simulink model "identifica_ip02"  (Simulink 7.2)
settings: Solver=ode4  StartTime=0.0  StopTime=10  FixedStep=0.001  RelTol=1e-3  AbsTol=1e-6
values from neighbouring files (symbols this model uses):
  Beq = 5.4    [matlab.mat]    (also in matlab2.mat)
  Eff_g = 1    [matlab.mat]    (also in matlab2.mat)
  Eff_m = 1    [matlab.mat]    (also in matlab2.mat)
  IMAX_AMP = 4    [matlab.mat]    (also in matlab2.mat)
  Jm = 3.90009575504e-07    [matlab.mat]    (also in matlab2.mat)
  K = yfinal*wn^2/amp_step    [estima_sys_2ordem.m]    (also in matlab.mat = 1; matlab2.mat = 1)
  K_AMP = 1    [matlab.mat]    (also in matlab2.mat)
  K_EC = 2.27485440932e-05    [matlab.mat]    (also in matlab2.mat)
  K_EP = 0.00153398078789    [matlab.mat]    (also in matlab2.mat)
  Kg = 3.71    [matlab.mat]    (also in matlab2.mat)
  Km = 0.00767763445475    [matlab.mat]    (also in matlab2.mat)
  Kt = 0.00768296972928    [matlab.mat]    (also in matlab2.mat)
  M = 0.94    [matlab.mat]    (also in matlab2.mat)
  qsi = -log(SP/100)/sqrt(pi^2+log(SP/100)^2)    [estima_sys_2ordem.m]    (also in matlab.mat = 1; matlab2.mat = 1)
  r_mp = 0.00635    [matlab.mat]    (also in matlab2.mat)
  R_SLEW_RATE = 500    [matlab.mat]    (also in matlab2.mat)
  Rm = 2.6    [matlab.mat]    (also in matlab2.mat)
  VMAX_AMP = 24    [matlab.mat]    (also in matlab2.mat)
  VMAX_DAC = 10    [matlab.mat]    (also in matlab2.mat)
  wn = pi/(Tp*sqrt(1-qsi^2))    [estima_sys_2ordem.m]    (also in identificacao.m = pi/(tp*sqrt(1-ksi^2)); matlab.mat = 1; matlab2.mat = 1)
  X_LIM_ENABLE = 1    [matlab.mat]    (also in matlab2.mat)
  X_MAX = 0.3    [matlab.mat]    (also in matlab2.mat)
  X_MIN = -0.3    [matlab.mat]    (also in matlab2.mat)
undefined symbols (not defined in the file or in its folder): HIL, qc_get_step_size
libraries: quarc_library x5, simulink x2, simulink_extras x1
CloseFcn:
  | rtwprivate ssgencode ModelCloseRequest q_position_pv_ip02
settings Model: Creator=Mfotoohi  LastModifiedBy=aluno  SimulationMode=external  ExtModeTrigDuration=50000  BufferReuse=off
settings SolverCC: PositivePriorityOrder=on
settings DataIOCC: LimitDataPoints=off
settings OptimizationCC: BooleanDataType=off  InlineInvariantSignals=on  OptimizeBlockIOStorage=off  BufferReuse=off  EnforceIntegerDowncast=off  ExpressionFolding=off  FoldNonRolledExpr=off  LocalBlockOutputs=off  InitFltsAndDblsToZero=on
settings DebuggingCC: SaveWithParameterizedLinksMsg=none  SignalResolutionControl=TryResolveAllWithWarning  SolverPrmCheckMsg=none  MultiTaskDSMMsg=warning  MultiTaskCondExecSysMsg=none  StrictBusMsg=None
settings HardwareCC: TargetHWDeviceType=32-bit Generic
settings RTWCC: SystemTargetFile=quarc_windows.tlc  TemplateMakefile=quarc_default_tmf  Description=Quarc Win32 Target  ProcessScript=quarc_windows_make_rtw_hook  IncludeERTFirstTime=on
settings STFCustomTargetCC: TargetFcnLib=ansi_tfl_tmw.mat  TargetPreCompLibLocation=C:\DOCUME~1\ALLUSE~1\DADOSD~1\QUARC\lib\2008b\windows\release  SystemTargetFile=quarc_windows.tlc
settings GRTTargetCC: TargetFcnLib=ansi_tfl_tmw.mat  TargetPreCompLibLocation=C:\DOCUME~1\ALLUSE~1\DADOSD~1\QUARC\lib\2008b\windows\release  CompOptLevelCompliant=off  MatFileLogging=off  ExtMode=on  ExtModeMexFile=quarc_comm

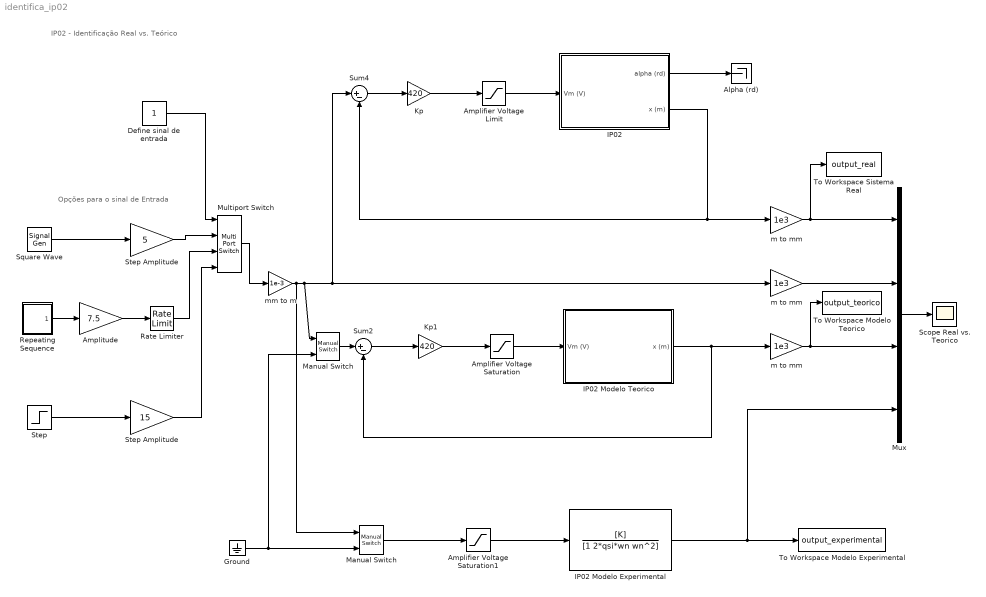
== system identifica_ip02 ==
  note: IP02 - Identificação
      | Real vs. Teórico
  note: Opções para o sinal de Entrada
  Alpha (rd) : Terminator
  Amplifier Voltage Limit : Saturate  UpperLimit=VMAX_AMP  LowerLimit=- VMAX_AMP
  Amplifier Voltage Saturation : Saturate  UpperLimit=VMAX_AMP  LowerLimit=- VMAX_AMP
  Amplifier Voltage Saturation1 : Saturate  UpperLimit=VMAX_AMP  LowerLimit=- VMAX_AMP
  Amplitude : Gain  Gain=7.5  ParameterDataType=sfix(16)  ParameterScaling=2^0  OutDataType=sfix(16)  OutScaling=2^0  SaturateOnIntegerOverflow=on  OutDataTypeStr=Inherit: Same as input  ParamDataTypeStr=Inherit: Same as input
  Define sinal de entrada : Constant  OutDataType=fixdt(1, 16)  OutScaling=2^0
  Ground : Ground
  IP02 : Subsystem
  IP02 Modelo Experimental : TransferFcn  Numerator=[K]  Denominator=[1 2*qsi*wn wn^2]
  IP02 Modelo Teorico : Subsystem
  Kp : Gain  Gain=420  ParameterDataType=sfix(16)  ParameterScaling=2^0  OutDataType=sfix(16)  OutScaling=2^0  SaturateOnIntegerOverflow=on  OutDataTypeStr=Inherit: Same as input  ParamDataTypeStr=Inherit: Same as input
  Kp1 : Gain  Gain=420  ParameterDataType=sfix(16)  ParameterScaling=2^0  OutDataType=sfix(16)  OutScaling=2^0  SaturateOnIntegerOverflow=on  OutDataTypeStr=Inherit: Same as input  ParamDataTypeStr=Inherit: Same as input
  Manual Switch : simulink/Signal Routing/Manual Switch  SystemSampleTime=-1  sw=0  action=0  varsize=off
  "Manual Switch " : simulink/Signal Routing/Manual Switch  SystemSampleTime=-1  sw=0  action=0  varsize=off
  Multiport Switch : MultiPortSwitch  OutDataType=fixdt(1, 16)  OutScaling=2^0
  Mux : Mux
  Rate Limiter : RateLimiter  RisingSlewLimit=R_SLEW_RATE  FallingSlewLimit=- R_SLEW_RATE
  Repeating Sequence : Subsystem  mask(Repeating table){@1=[0 10 10 30 30  50 ]*0.2, @2=[0 0 1 1 -1 -1]}
      mask prompts: @1 "Time values:"; @2 "Output values:"
      mask help:
      | Repeating table.
      | Enter values of time and output for first cycle.
      mask init:
      | period = max(@1); t = @1; y = @2;
      mask Help: Repeats cycle given in table. Time values should be monotonically increasing.
      mask Display: plot([t,t+period,t+2*period],[y,y,y])
  Scope Real vs. Teorico : Scope
      settings: TickLabels=on  TimeRange=5  YMin=-11  YMax=11  SaveName=x  DataFormat=Array
  Square Wave : SignalGenerator  WaveForm=square  Frequency=0.66
  Step : Step  Time=0  SampleTime=0
  Step Amplitude : Gain  Gain=5  ParameterDataType=sfix(16)  ParameterScaling=2^0  OutDataType=sfix(16)  OutScaling=2^0  SaturateOnIntegerOverflow=on  OutDataTypeStr=Inherit: Same as input  ParamDataTypeStr=Inherit: Same as input
  "Step Amplitude " : Gain  Gain=15  ParameterDataType=sfix(16)  ParameterScaling=2^0  OutDataType=sfix(16)  OutScaling=2^0  SaturateOnIntegerOverflow=on  OutDataTypeStr=Inherit: Same as input  ParamDataTypeStr=Inherit: Same as input
  Sum2 : Sum  Inputs=|+-  OutDataType=sfix(16)  OutScaling=2^0  SaturateOnIntegerOverflow=on  InputSameDT=on  OutDataTypeStr=Inherit: Same as first input
  Sum4 : Sum  Inputs=|+-  OutDataType=sfix(16)  OutScaling=2^0  SaturateOnIntegerOverflow=on  InputSameDT=on  OutDataTypeStr=Inherit: Same as first input
  To Workspace Modelo Experimental : ToWorkspace  VariableName=output_experimental  SampleTime=-1  SaveFormat=Structure With Time
  To Workspace Modelo Teorico : ToWorkspace  VariableName=output_teorico  SampleTime=-1  SaveFormat=Structure With Time
  To Workspace Sistema Real : ToWorkspace  VariableName=output_real  SampleTime=-1  SaveFormat=Structure With Time
  m to mm : Gain  Gain=1e3  ParameterDataType=sfix(16)  ParameterScaling=2^0  OutDataType=sfix(16)  OutScaling=2^0  SaturateOnIntegerOverflow=on  OutDataTypeStr=Inherit: Same as input  ParamDataTypeStr=Inherit: Same as input
  "m to mm " : Gain  Gain=1e3  ParameterDataType=sfix(16)  ParameterScaling=2^0  OutDataType=sfix(16)  OutScaling=2^0  SaturateOnIntegerOverflow=on  OutDataTypeStr=Inherit: Same as input  ParamDataTypeStr=Inherit: Same as input
  "m to mm  " : Gain  Gain=1e3  ParameterDataType=sfix(16)  ParameterScaling=2^0  OutDataType=sfix(16)  OutScaling=2^0  SaturateOnIntegerOverflow=on  OutDataTypeStr=Inherit: Same as input  ParamDataTypeStr=Inherit: Same as input
  mm to m : Gain  Gain=1e-3  ParameterDataType=sfix(16)  ParameterScaling=2^0  OutDataType=sfix(16)  OutScaling=2^0
  wires:
  Sum2/1 -> Kp1/1
  IP02/2(x (m)) -> m to mm/1, Sum4/2
  IP02 Modelo Teorico/1(x (m)) -> "m to mm  "/1, Sum2/2
  Sum4/1 -> Kp/1
  Kp1/1 -> Amplifier Voltage Saturation/1
  Amplifier Voltage Saturation/1 -> IP02 Modelo Teorico/1(Vm (V))
  Mux/1 -> Scope Real vs. Teorico/1
  Repeating Sequence/1(out_1) -> Amplitude/1
  Amplifier Voltage Limit/1 -> IP02/1(Vm (V))
  IP02/1(alpha (rd)) -> Alpha (rd)/1
  Step Amplitude/1 -> Multiport Switch/2
  Amplitude/1 -> Rate Limiter/1
  Rate Limiter/1 -> Multiport Switch/3
  Kp/1 -> Amplifier Voltage Limit/1
  mm to m/1 -> Manual Switch/1, Sum4/1, "m to mm "/1, "Manual Switch "/1
  Define sinal de entrada/1 -> Multiport Switch/1
  "Step Amplitude "/1 -> Multiport Switch/4
  Step/1 -> "Step Amplitude "/1
  IP02 Modelo Experimental/1 -> Mux/4, To Workspace Modelo Experimental/1
  Amplifier Voltage Saturation1/1 -> IP02 Modelo Experimental/1
  m to mm/1 -> To Workspace Sistema Real/1, Mux/1
  "m to mm "/1 -> Mux/2
  "m to mm  "/1 -> Mux/3, To Workspace Modelo Teorico/1
  Square Wave/1 -> Step Amplitude/1
  Multiport Switch/1 -> mm to m/1
  Manual Switch/1 -> Amplifier Voltage Saturation1/1
  Ground/1 -> Manual Switch/2, "Manual Switch "/2
  "Manual Switch "/1 -> Sum2/1

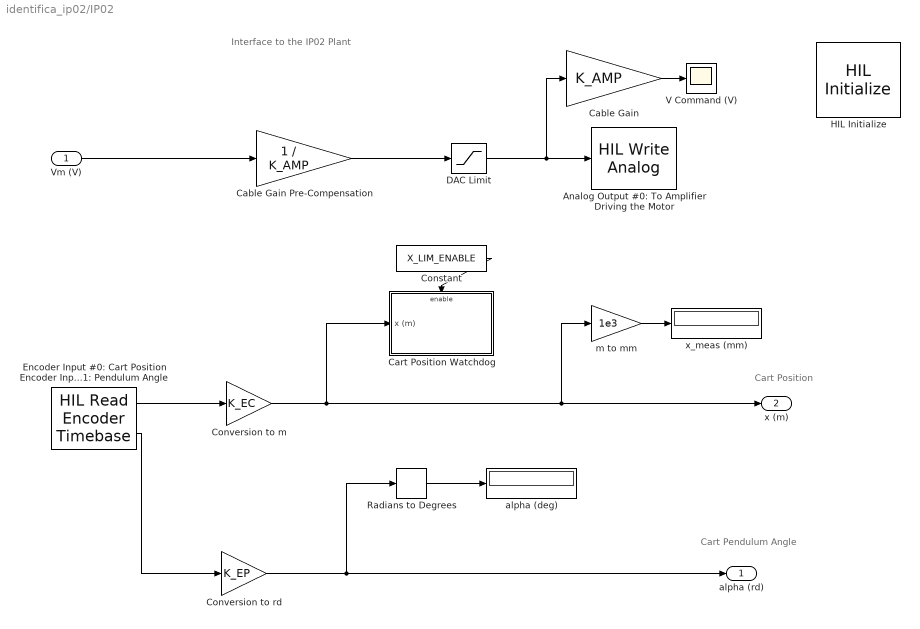
== system identifica_ip02/IP02 ==
  note: Cart Pendulum Angle
  note: Cart Position
  note: Interface to the IP02 Plant
  Vm (V) : Inport  OutDataType=sfix(16)  OutScaling=2^0
  Analog Output #0: To Amplifier Driving the Motor : quarc_library/Data Acquisition/Generic/Immediate I//O/HIL Write Analog  Tag=unassigned  object_name=HIL-1  channels=0  sample_time=-1  active=on  vector_input=on
  Cable Gain : Gain  Gain=K_AMP  ParameterDataType=sfix(16)  ParameterScaling=2^0  OutDataType=sfix(16)  OutScaling=2^0  SaturateOnIntegerOverflow=on  OutDataTypeStr=Inherit: Same as input  ParamDataTypeStr=Inherit: Same as input
  Cable Gain Pre-Compensation : Gain  Gain=1 / K_AMP  ParameterDataType=sfix(16)  ParameterScaling=2^0  OutDataType=sfix(16)  OutScaling=2^0  SaturateOnIntegerOverflow=on  OutDataTypeStr=Inherit: Same as input  ParamDataTypeStr=Inherit: Same as input
  Cart Position Watchdog : Subsystem  TreatAsAtomicUnit=on
  Constant : Constant  Value=X_LIM_ENABLE  OutDataType=sfix(16)  OutScaling=2^0
  Conversion to m : Gain  Gain=K_EC  ParameterDataType=sfix(16)  ParameterScaling=2^0  OutDataType=sfix(16)  OutScaling=2^0  SaturateOnIntegerOverflow=on  OutDataTypeStr=Inherit: Same as input  ParamDataTypeStr=Inherit: Same as input
  Conversion to rd : Gain  Gain=K_EP  ParameterDataType=sfix(16)  ParameterScaling=2^0  OutDataType=sfix(16)  OutScaling=2^0  SaturateOnIntegerOverflow=on  OutDataTypeStr=Inherit: Same as input  ParamDataTypeStr=Inherit: Same as input
  DAC Limit : Saturate  UpperLimit=VMAX_DAC  LowerLimit=- VMAX_DAC
  Encoder Input #0: Cart Position Encoder Input #1: Pendulum Angle : quarc_library/Data Acquisition/Generic/Timebases/HIL Read Encoder Timebase  Tag=unassigned  object_name=HIL-1  clock=0  channels=[0,1]  samples_in_buffer=max(ceil(1/qc_get_step_size), 1)  active=on  vector_output=off  data_type_mode=Inherit via back propagation  data_type=double
  HIL Initialize : quarc_library/Data Acquisition/Generic/Configuration/HIL Initialize  object_name=HIL-1  board_type=q8_usb  board_number=0  board_options=update_rate=normal  exclusive=off  active=off  hardware_clocks=[0:2]  clock_modes=[]  set_clock_params_at_start=off  set_clock_params_at_switch_in=off  analog_input_channels=[0:7]  analog_input_maximums=10  analog_input_minimums=-10  set_analog_input_params_at_start=on  set_analog_input_params_at_switch_in=off  analog_output_channels=[0:7]  analog_output_maximums=10  analog_output_minimums=-10  initial_analog_outputs=[0]  final_analog_outputs=[0]  watchdog_analog_outputs=0  set_analog_output_params_at_start=on  set_analog_output_params_at_switch_in=off  set_analog_outputs_at_start=on  set_analog_outputs_at_switch_in=off  set_analog_outputs_at_terminate=on  set_analog_outputs_at_switch_out=off  set_analog_outputs_on_watchdog=off  digital_input_channels=[]  digital_output_channels=[0:7]  digital_output_configuration=[]  initial_digital_outputs=[0]  final_digital_outputs=[0]  watchdog_digital_outputs=[0]  set_digital_output_params_at_start=off  set_digital_output_params_at_switch_in=off  set_digital_outputs_at_start=on  set_digital_outputs_at_switch_in=off  set_digital_outputs_at_terminate=on  set_digital_outputs_at_switch_out=off  set_digital_outputs_on_watchdog=off  encoder_channels=[0:7]  quadrature=[4]  encoder_filter_frequency=[]  initial_encoder_counts=[0]  set_encoder_params_at_start=on  set_encoder_params_at_switch_in=off  set_encoder_counts_at_start=on  set_encoder_counts_at_switch_in=off  pwm_channels=[0:7]  pwm_modes=0  pwm_frequency=99.532799999999995e6/4095  pwm_configuration=[0]  pwm_alignment=[0]  pwm_polarity=[1]  pwm_leading_deadband=[0]  pwm_trailing_deadband=[0]  initial_pwm_outputs=[0]  final_pwm_outputs=[0]  watchdog_pwm_outputs=[0]  set_pwm_params_at_start=on  set_pwm_params_at_switch_in=off  set_pwm_outputs_at_start=on  set_pwm_outputs_at_switch_in=off  set_pwm_outputs_at_terminate=on  set_pwm_outputs_at_switch_out=off  set_pwm_outputs_on_watchdog=off  other_output_channels=[]  initial_other_outputs=[]  final_other_outputs=[]  watchdog_other_outputs=[]  set_other_outputs_at_start=off  set_other_outputs_at_switch_in=off  set_other_outputs_at_terminate=off  set_other_outputs_at_switch_out=off  set_other_outputs_on_watchdog=off
  Radians to Degrees : simulink_extras/Transformations/Radians to Degrees  SystemSampleTime=-1
  V Command (V) : Scope
      settings: TickLabels=on  TimeRange=5  YMin=-3  YMax=2.5  SaveName=data_vm  DataFormat=Array  MaxDataPoints=2500
  alpha (deg) : Display
      settings: Decimation=100
  m to mm : Gain  Gain=1e3  ParameterDataType=sfix(16)  ParameterScaling=2^0  OutDataType=sfix(16)  OutScaling=2^0  SaturateOnIntegerOverflow=on  OutDataTypeStr=Inherit: Same as input  ParamDataTypeStr=Inherit: Same as input
  x_meas (mm) : Display
      settings: Decimation=100
  alpha (rd) : Outport  OutDataType=sfix(16)  OutScaling=2^0  InitialOutput=0
  x (m) : Outport  Port=2  OutDataType=sfix(16)  OutScaling=2^0  InitialOutput=0
  wires:
  Encoder Input #0: Cart Position Encoder Input #1: Pendulum Angle/1 -> Conversion to m/1
  Conversion to m/1 -> Cart Position Watchdog/1(x (m)), x (m)/1, m to mm/1
  Cable Gain Pre-Compensation/1 -> DAC Limit/1
  m to mm/1 -> x_meas (mm)/1
  Encoder Input #0: Cart Position Encoder Input #1: Pendulum Angle/2 -> Conversion to rd/1
  Radians to Degrees/1 -> alpha (deg)/1
  Conversion to rd/1 -> Radians to Degrees/1, alpha (rd)/1
  Constant/1 -> Cart Position Watchdog/Enable
  DAC Limit/1 -> Analog Output #0: To Amplifier Driving the Motor/1, Cable Gain/1
  Vm (V)/1 -> Cable Gain Pre-Compensation/1
  Cable Gain/1 -> V Command (V)/1

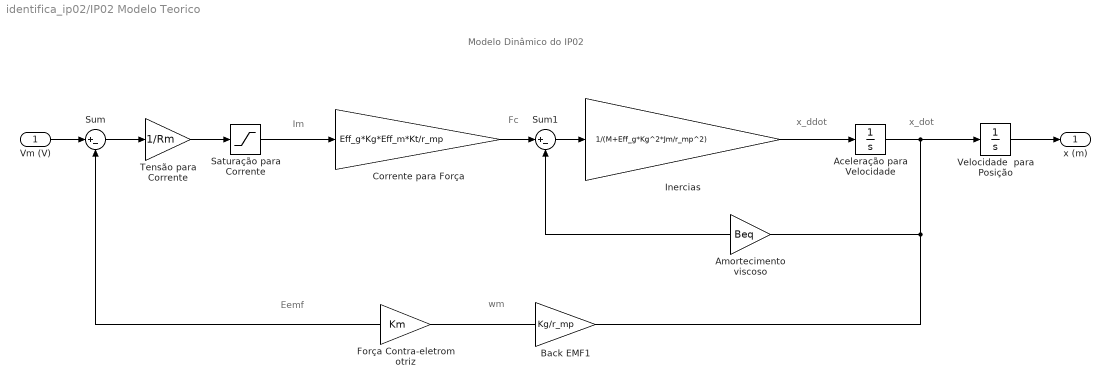
== system identifica_ip02/IP02 Modelo Teorico ==
  note: Modelo Dinâmico do IP02
  note: Fc
  note: Im
  note: Eemf
  note: wm
  note: x_dot
  note: x_ddot
  Vm (V) : Inport  OutDataType=sfix(16)  OutScaling=2^0
  Aceleração para Velocidade : Integrator
  Amortecimento viscoso : Gain  Gain=Beq  ParameterDataType=sfix(16)  ParameterScaling=2^0  OutDataType=sfix(16)  OutScaling=2^0  SaturateOnIntegerOverflow=on  OutDataTypeStr=Inherit: Same as input  ParamDataTypeStr=Inherit: Same as input
  Back EMF1 : Gain  Gain=Kg/r_mp  ParameterDataType=sfix(16)  ParameterScaling=2^0  OutDataType=sfix(16)  OutScaling=2^0  SaturateOnIntegerOverflow=on  OutDataTypeStr=Inherit: Same as input  ParamDataTypeStr=Inherit: Same as input
  Corrente para Força : Gain  Gain=Eff_g*Kg*Eff_m*Kt/r_mp  ParameterDataType=sfix(16)  ParameterScaling=2^0  OutDataType=sfix(16)  OutScaling=2^0  SaturateOnIntegerOverflow=on  OutDataTypeStr=Inherit: Same as input  ParamDataTypeStr=Inherit: Same as input
  Força Contra-eletromotriz : Gain  Gain=Km  ParameterDataType=sfix(16)  ParameterScaling=2^0  OutDataType=sfix(16)  OutScaling=2^0  SaturateOnIntegerOverflow=on  OutDataTypeStr=Inherit: Same as input  ParamDataTypeStr=Inherit: Same as input
  Inercias : Gain  Gain=1/(M+Eff_g*Kg^2*Jm/r_mp^2)  ParameterDataType=sfix(16)  ParameterScaling=2^0  OutDataType=sfix(16)  OutScaling=2^0  SaturateOnIntegerOverflow=on  OutDataTypeStr=Inherit: Same as input  ParamDataTypeStr=Inherit: Same as input
  Saturação para Corrente : Saturate  UpperLimit=IMAX_AMP  LowerLimit=- IMAX_AMP
  Sum : Sum  Inputs=|+-  OutDataType=sfix(16)  OutScaling=2^0  SaturateOnIntegerOverflow=on  InputSameDT=on  OutDataTypeStr=Inherit: Same as first input
  Sum1 : Sum  Inputs=|+-  OutDataType=sfix(16)  OutScaling=2^0  SaturateOnIntegerOverflow=on  InputSameDT=on  OutDataTypeStr=Inherit: Same as first input
  Tensão para Corrente : Gain  Gain=1/Rm  ParameterDataType=sfix(16)  ParameterScaling=2^0  OutDataType=sfix(16)  OutScaling=2^0  SaturateOnIntegerOverflow=on  OutDataTypeStr=Inherit: Same as input  ParamDataTypeStr=Inherit: Same as input
  Velocidade  para Posição : Integrator
  x (m) : Outport  OutDataType=sfix(16)  OutScaling=2^0
  wires:
  Sum/1 -> Tensão para Corrente/1
  Inercias/1 -> Aceleração para Velocidade/1
  Sum1/1 -> Inercias/1
  Tensão para Corrente/1 -> Saturação para Corrente/1
  Aceleração para Velocidade/1 -> Velocidade  para Posição/1, Back EMF1/1, Amortecimento viscoso/1
  Back EMF1/1 -> Força Contra-eletromotriz/1
  Saturação para Corrente/1 -> Corrente para Força/1
  Vm (V)/1 -> Sum/1
  Velocidade  para Posição/1 -> x (m)/1
  Corrente para Força/1 -> Sum1/1
  Amortecimento viscoso/1 -> Sum1/2
  Força Contra-eletromotriz/1 -> Sum/2

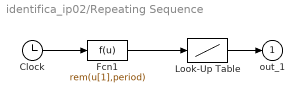
== system identifica_ip02/Repeating Sequence ==
  Clock : Clock
      settings: Decimation=10
  Fcn1 : Fcn  Expr=rem(u[1],period)
  Look-Up Table : Lookup  InputValues=t  Table=y  OutDataType=sfix(16)  OutScaling=2^0  SaturateOnIntegerOverflow=on
  out_1 : Outport  OutDataType=sfix(16)  OutScaling=2^0  InitialOutput=0
  wires:
  Look-Up Table/1 -> out_1/1
  Clock/1 -> Fcn1/1
  Fcn1/1 -> Look-Up Table/1

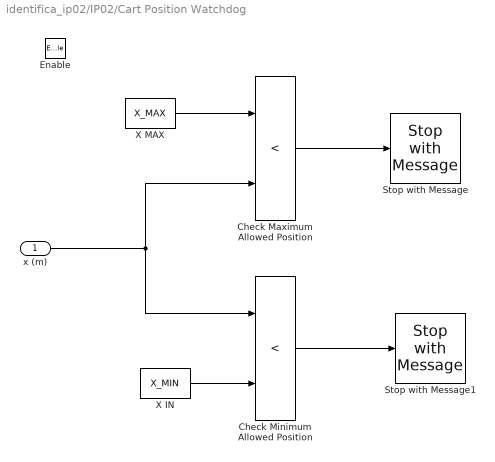
== system identifica_ip02/IP02/Cart Position Watchdog ==
  x (m) : Inport  OutDataType=sfix(16)  OutScaling=2^0
  Enable : EnablePort
  Check Maximum Allowed Position : RelationalOperator  Operator=<  InputSameDT=on
  Check Minimum Allowed Position : RelationalOperator  Operator=<  InputSameDT=on
  Stop with Message : quarc_library/Sinks/Error Handling/Stop with Message  SystemSampleTime=-1  message_type=Fixed error message  message_icon=Error  message=Maximum Limit Reached.
  Stop with Message1 : quarc_library/Sinks/Error Handling/Stop with Message  SystemSampleTime=-1  message_type=Fixed error message  message_icon=Error  message=Minimum Limit Reached.
  X IN : Constant  Value=X_MIN  OutDataType=sfix(16)  OutScaling=2^0
  X MAX : Constant  Value=X_MAX  OutDataType=sfix(16)  OutScaling=2^0
  wires:
  Check Maximum Allowed Position/1 -> Stop with Message/1
  x (m)/1 -> Check Minimum Allowed Position/1, Check Maximum Allowed Position/2
  X IN/1 -> Check Minimum Allowed Position/2
  Check Minimum Allowed Position/1 -> Stop with Message1/1
  X MAX/1 -> Check Maximum Allowed Position/1
